simulink model "MuxDemux"  (R2020a)
settings: Solver=VariableStepAuto  StartTime=0.0  StopTime=10.0  RelTol=1e-3
settings Model: Creator=royde  LastModifiedBy=royde

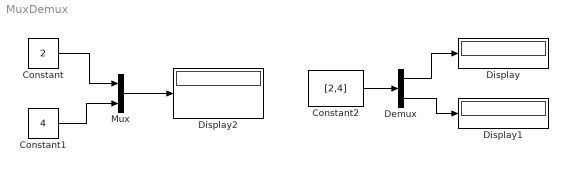
== system MuxDemux ==
  Constant : Constant  Value=2
  Constant1 : Constant  Value=4
  Constant2 : Constant  Value=[2,4]
  Demux : Demux  Outputs=2
  Display : Display
  Display1 : Display
  Display2 : Display
  Mux : Mux  Inputs=2
  wires:
  Constant/1 -> Mux/1
  Constant1/1 -> Mux/2
  Demux/1 -> Display/1
  Demux/2 -> Display1/1
  Mux/1 -> Display2/1
  Constant2/1 -> Demux/1
